simulink model "subsysNavigation"  (R2023b)
settings: Solver=VariableStepAuto  StartTime=0.0  StopTime=10.0  RelTol=1e-3
settings Model: Creator=neham  LastModifiedBy=neham

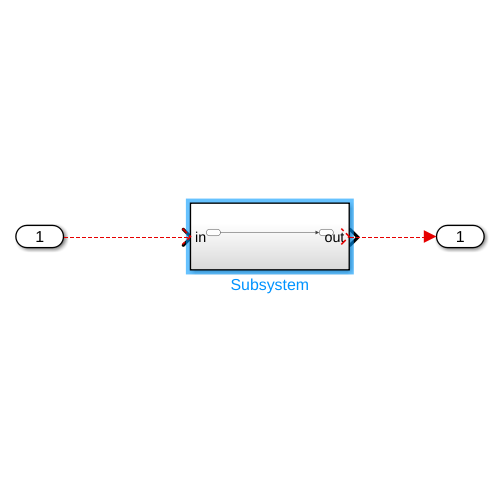
[thumbnail: Simulink's stored preview of the top-level diagram]
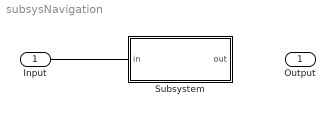
== system subsysNavigation ==
  Input : Inport
  Subsystem : Subsystem
  Output : Outport
  wires:
  Input/1 -> ?
  ? -> Output/1

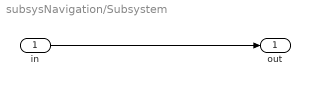
== system subsysNavigation/Subsystem ==
  in : Inport
  out : Outport
  wires:
  in/1 -> out/1
